simulink model "SMC_TwoLink"  (R2020b)
settings: Solver=VariableStepAuto  StartTime=0.0  StopTime=20  RelTol=1e-3
settings Model: Creator=MR.co  LastModifiedBy=MR.co

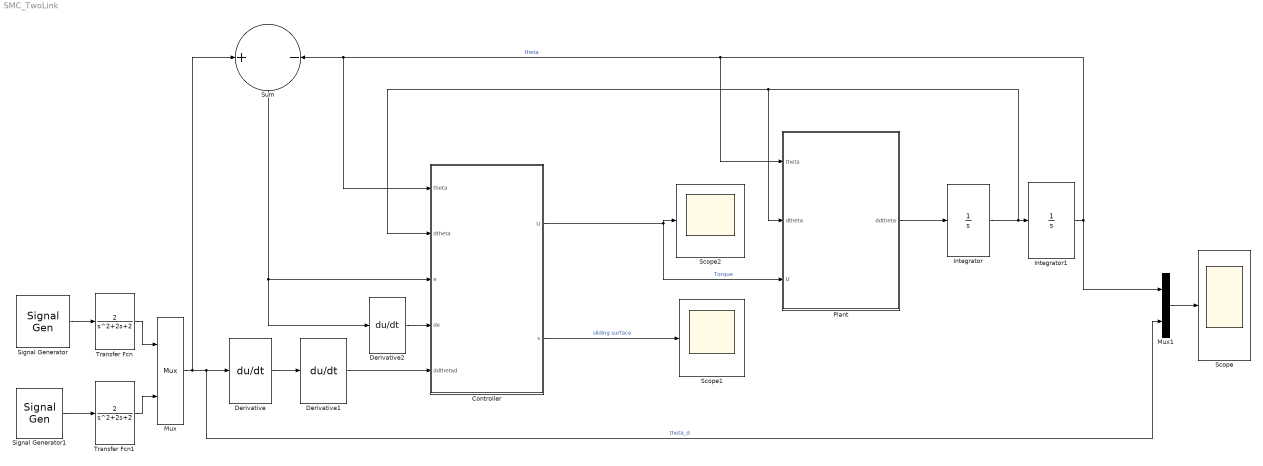
== system SMC_TwoLink ==
  Controller : MATLAB Function  TreatAsAtomicUnit=on
  Derivative : Derivative
  Derivative1 : Derivative
  Derivative2 : Derivative
  Integrator : Integrator  InitialCondition=zeros(2,1)
  Integrator1 : Integrator  InitialCondition=randn(2,1)
  Mux : Mux  Inputs=2
  Mux1 : Mux  Inputs=2
  Plant : MATLAB Function  TreatAsAtomicUnit=on
  Scope : Scope
  Scope1 : Scope
  Scope2 : Scope
  Signal Generator : SignalGenerator  Amplitude=2  Frequency=pi  Units=rad/sec
  Signal Generator1 : SignalGenerator  WaveForm=square  Amplitude=3  Frequency=pi/2  Units=rad/sec
  Sum : Sum  Inputs=+|-
  Transfer Fcn : TransferFcn  Numerator=[2]  Denominator=[1 2 2]
  Transfer Fcn1 : TransferFcn  Numerator=[2]  Denominator=[1 2 2]
  wires:
  Controller/1(U) -> Plant/3(U), Scope2/1  "Torque"
  Plant/1(ddtheta) -> Integrator/1
  Integrator/1 -> Plant/2(dtheta), Controller/2(dtheta), Integrator1/1
  Signal Generator/1 -> Transfer Fcn/1
  Signal Generator1/1 -> Transfer Fcn1/1
  Transfer Fcn1/1 -> Mux/2
  Transfer Fcn/1 -> Mux/1
  Derivative/1 -> Derivative1/1
  Derivative1/1 -> Controller/5(ddthetad)
  Integrator1/1 -> Mux1/1, Plant/1(theta), Sum/2, Controller/1(theta)  "theta"
  Mux/1 -> Mux1/2, Derivative/1, Sum/1  "theta_d"
  Sum/1 -> Derivative2/1, Controller/3(e)
  Derivative2/1 -> Controller/4(de)
  Mux1/1 -> Scope/1
  Controller/2(s) -> Scope1/1  "sliding surface"

== matlab function SMC_TwoLink/Controller ==
  data: theta input; U output; dtheta input; e input; de input; ddthetad input; s output
function [U , s]= fcn( theta , dtheta , e , de, ddthetad)


    L1 = 1; % m
    L2 = 1.2; % m
    
    Lc1 = .5; % m
    Lc2 = .6; % m
     
    m1 = 1; % Kg
    m2 = 2; % Kg
    
    I1 = 1/12 * m1 * L1^2;  %kg.N
    I2 = 1/12 * m2 * L2^2;  %kg.N

    g = 9.8; % m/s^2
   
    
    M11 = m1 * Lc1^2 + I1 + m2*(L1^2 + Lc2^2 + 2 * L1 * Lc2 * cos(theta(2))) + I2;
    M12 = m2 * L1 * Lc2 * cos(theta(2)) + m2 * Lc2^2 + I2;
    M22 = m2 * Lc2^2 + I2;
    M=[M11 M12;M12 M22];

    G1 = m1 * Lc1 * cos(theta(1)) + m2 * (Lc2 * cos(theta(1) + theta(2)) + L1 * cos(theta(1)));
    G2 = m2 * Lc2 * cos(theta(1) + theta(2));
    G=[G1*g;G2*g];
    
    F12 = m2 * L1 * Lc2 * sin(theta(2));
    C=[-F12*dtheta(2) -F12*(dtheta(1)+dtheta(2));F12*dtheta(1) 0];
  
    c =  8 * eye(2);
    ebs = 8 * eye(2);
    s = de + c * e;
   
    U = M * (ddthetad + c* de + ebs * sign(s)) + C * dtheta + G;

== matlab function SMC_TwoLink/Plant ==
  data: theta input; ddtheta output; dtheta input; U input
function ddtheta = fcn( theta , dtheta , U)


    L1 = 1; % m
    L2 = 1.2; % m
    
    Lc1 = .5; % m
    Lc2 = .6; % m
     
    m1 = 1; % Kg
    m2 = 2; % Kg
    
    I1 = 1/12 * m1 * L1^2;  %kg.N
    I2 = 1/12 * m2 * L2^2;  %kg.N

    g = 9.8; % m/s^2
   
    
    M11 = m1 * Lc1^2 + I1 + m2*(L1^2 + Lc2^2 + 2 * L1 * Lc2 * cos(theta(2))) + I2;
    M12 = m2 * L1 * Lc2 * cos(theta(2)) + m2 * Lc2^2 + I2;
    M22 = m2 * Lc2^2 + I2;
    M=[M11 M12;M12 M22];

    G1 = m1 * Lc1 * cos(theta(1)) + m2 * (Lc2 * cos(theta(1) + theta(2)) + L1 * cos(theta(1)));
    G2 = m2 * Lc2 * cos(theta(1) + theta(2));
    G=[G1*g;G2*g];
    
    F12 = m2 * L1 * Lc2 * sin(theta(2));
    C=[-F12*dtheta(2) -F12*(dtheta(1)+dtheta(2));F12*dtheta(1) 0];
    
    
    ddtheta = M\( U -C*dtheta -G );
